simulink model "noHysteresisFastSlow"  (R2015b)
settings: Solver=ode45  StartTime=0.0  StopTime=20  RelTol=1e-3
values from neighbouring files (symbols this model uses):
  alpha_const = 0.0    (= 0)    [averagedRelayOutput.m]    (also in bursting_linearised.m = 0.1; fastSlow.m; manParamsNullclines.m; manipulateParameters.m = getappdata(hObject.Parent,'alpha_const'))
  beta = 0.37    [averagedRelayOutput.m]    (also in bursting_linearised.m = 0.27; compareApproximations.m = 1.5; fastSlow.m; fast_nullcline_winged_cusp.m = 0.5)
  gamma = 0    [averagedRelayOutput.m]    (also in bursting_linearised.m = 1; compareApproximations.m = 1; fastSlow.m; fast_nullcline_winged_cusp.m = 1)
  slow_plant_X0 = -1.0    (= -1)    [averagedRelayOutput.m]    (also in bursting_linearised.m = -1.05; fastSlow.m; fast_nullcline_winged_cusp.m = -1.05; hRose.m = -10)
  ts = 1    [averagedRelayOutput.m]    (also in bursting_linearised.m; compareApproximations.m; fastSlow.m; fast_nullcline_winged_cusp.m)
  tus = 800    [averagedRelayOutput.m]    (also in bursting_linearised.m; fastSlow.m; manParamsNullclines.m; manipulateParameters.m = getappdata(hObject.Parent,'tus'))
  ultra_slow_plant_X0 = 0.45    [averagedRelayOutput.m]    (also in bursting_linearised.m = 0; fastSlow.m; hRose.m = 2000; manParamsNullclines.m)
settings Model: Creator=ra428  LastModifiedBy=rajiv
settings DataIOCC: SaveFormat=Array
settings HardwareCC: ProdBitPerPointer=32  ProdLargestAtomicFloat=None  ProdIntDivRoundTo=Undefined  ProdEndianess=Unspecified  ProdWordSize=32  ProdHWDeviceType=32-bit Generic
settings GRTTargetCC: GeneratePreprocessorConditionals=Disable all
settings ConfigComp: CovModelRefEnable=Off

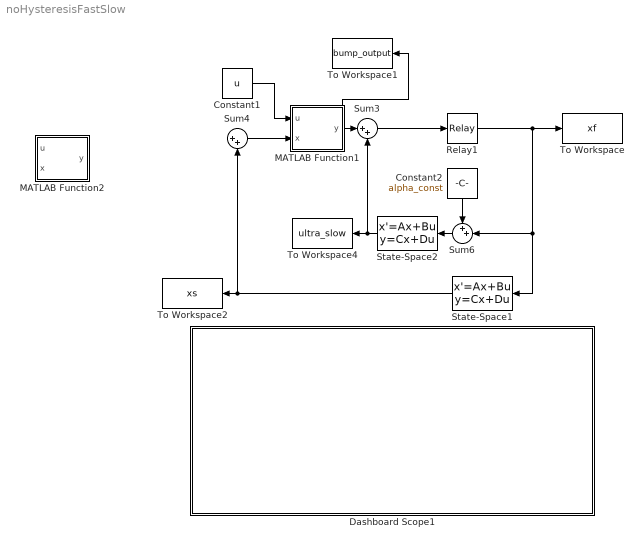
== system noHysteresisFastSlow ==
  Constant1 : Constant  Value=u
  Constant2 : Constant  Value=alpha_const
  Dashboard Scope1 : Subsystem  DialogController=hmiCreateDDGDialog  IsWebBlock=on  mask(MathWorksWebBlock){webBlockId=79cba157-b437-4935-ab1f-1ad6ca43220e, webBlockType=sdiscope, ShowInitialText=on, HMISrcModelName=noHysteresisFastSlow}
      mask prompts: webBlockId "WebBlock Id"; webBlockType "WebBlock Type"; HMISrcModelName "Source Model"
      mask Help: helpview([docroot '/mapfiles/simulink.map'], 'hmi_scope')
      mask Display:
      | if strcmp(get_param(bdroot(gcb),'BlockDiagramType'), 'library')
      |     image([(matlabroot) '/toolbox/simulink/hmi/icons/DashboardScope.png']);
      | end
  MATLAB Function1 : MATLAB Function  TreatAsAtomicUnit=on
  MATLAB Function2 : MATLAB Function  TreatAsAtomicUnit=on
  Relay1 : Relay  OnSwitchValue=beta  OffSwitchValue=-beta  OffOutputValue=-1
  State-Space1 : StateSpace  A=-1/ts  B=1/ts  D=0.5*1*gamma  X0=slow_plant_X0
  State-Space2 : StateSpace  A=-1/tus  B=-1/tus  D=0  X0=ultra_slow_plant_X0
  Sum3 : Sum  Inputs=|++
  Sum4 : Sum  Inputs=|++
  Sum6 : Sum  Inputs=++|
  To Workspace : ToWorkspace  VariableName=xf  SaveFormat=Timeseries  SampleTime=-1
  To Workspace1 : ToWorkspace  VariableName=bump_output  SaveFormat=Timeseries  SampleTime=-1
  To Workspace2 : ToWorkspace  VariableName=xs  SaveFormat=Timeseries  SampleTime=-1
  To Workspace4 : ToWorkspace  VariableName=ultra_slow  SaveFormat=Timeseries  SampleTime=-1
  wires:
  Sum3/1 -> Relay1/1
  Constant1/1 -> MATLAB Function1/1(u)
  Relay1/1 -> Sum6/2, State-Space1/1, To Workspace/1
  State-Space1/1 -> Sum4/2, To Workspace2/1
  Constant2/1 -> Sum6/1
  Sum6/1 -> State-Space2/1
  Sum4/1 -> MATLAB Function1/2(x)
  MATLAB Function1/1(y) -> To Workspace1/1, Sum3/1
  State-Space2/1 -> To Workspace4/1, Sum3/2

== system noHysteresisFastSlow/Dashboard Scope1 ==

== matlab function noHysteresisFastSlow/MATLAB Function1 ==
  data: u input; x input; y output
function y = fcn(u,x)
%#codegen
if (x < -2-u)
    y = 0;
elseif (x > 2-u)
    y = -1;
elseif and( x>=-2-u,x < -u)
    y = 0;
else
    y = -0.5*(x+u);
end

== matlab function noHysteresisFastSlow/MATLAB Function2 ==
  data: u input; x input; y output
function y = fcn(u,x)
%#codegen
if (x < -2-u)
    y = -1;
elseif (x > 2-u)
    y = -1;
elseif and( x>=-2-u,x < -u)
    y = 0.5*(x+u);
else
    y = -0.5*(x+u);
end
